simulink model "modelagem_controle_pratica3"  (R2023a)
settings: Solver=VariableStepAuto  StartTime=0.0  StopTime=10.0  RelTol=1e-3
model workspace (MAT data in the model file):
  B = 0.1
  J = 0.01
  Ke = 0.01
  Kt = 0.01
  L = 0.5
  R = 1
settings Model: Creator=Alexandre  LastModifiedBy=Alexandre

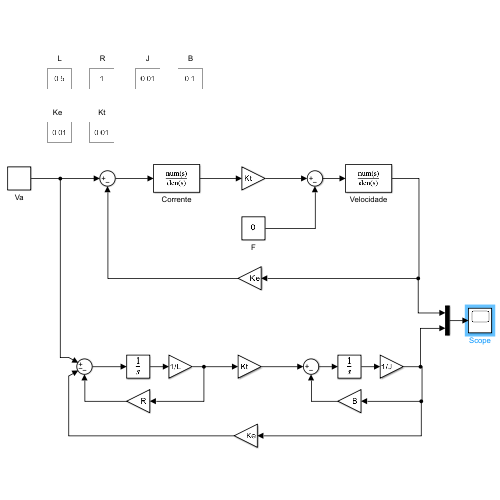
[thumbnail: Simulink's stored preview of the top-level diagram]
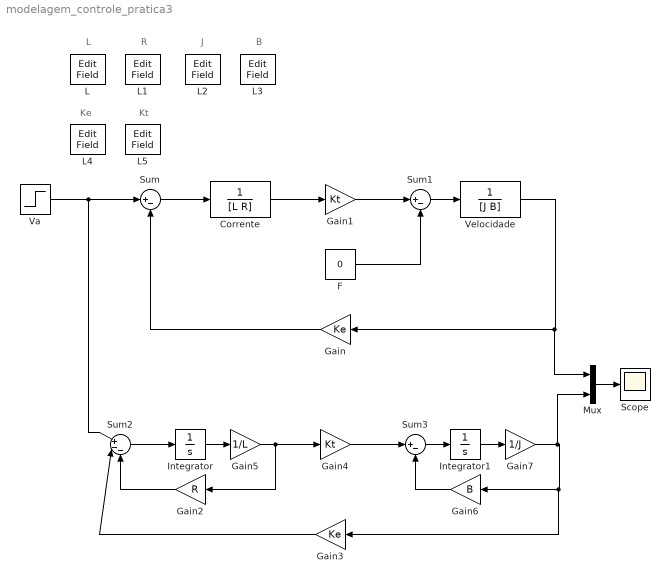
== system modelagem_controle_pratica3 ==
  note: J
  note: Kt
  note: Ke
  note: B
  note: L
  note: R
  Corrente : TransferFcn  Denominator=[L R]
  F : Constant  Value=0
  Gain : Gain  Gain=Ke
  Gain1 : Gain  Gain=Kt
  Gain2 : Gain  Gain=R
  Gain3 : Gain  Gain=Ke
  Gain4 : Gain  Gain=Kt
  Gain5 : Gain  Gain=1/L
  Gain6 : Gain  Gain=B
  Gain7 : Gain  Gain=1/J
  Integrator : Integrator
  Integrator1 : Integrator
  L{,1..5} (6 alike) : EditField  LabelPosition=Hide  ShowInitialText=on  Alignment=Center
  Mux : Mux  Inputs=2
  Scope : Scope
  Sum : Sum  Inputs=|+-
  Sum1 : Sum  Inputs=|+-
  Sum2 : Sum  Inputs=|+--
  Sum3 : Sum  Inputs=|+-
  Va : Step  Time=0  After=5  SampleTime=0
  Velocidade : TransferFcn  Denominator=[J B]
  wires:
  Sum/1 -> Corrente/1
  Velocidade/1 -> Mux/1, Gain/1
  Corrente/1 -> Gain1/1
  Va/1 -> Sum/1, Sum2/1
  Gain1/1 -> Sum1/1
  Gain/1 -> Sum/2
  F/1 -> Sum1/2
  Sum1/1 -> Velocidade/1
  Sum2/1 -> Integrator/1
  Gain2/1 -> Sum2/3
  Integrator/1 -> Gain5/1
  Gain3/1 -> Sum2/2
  Gain4/1 -> Sum3/1
  Sum3/1 -> Integrator1/1
  Gain5/1 -> Gain2/1, Gain4/1
  Gain6/1 -> Sum3/2
  Integrator1/1 -> Gain7/1
  Gain7/1 -> Mux/2, Gain3/1, Gain6/1
  Mux/1 -> Scope/1
